simulink model "test"  (R2015b)
settings: Solver=VariableStepAuto  StartTime=0.0  StopTime=10.0  RelTol=1e-3
undefined symbols (not defined in the file or in its folder): etaCmax, etaCmin, m_dot_cCorr, PiC, PiC_at_etaCmax, Q11, Q12, Q22, WcCorr_at_etaCmax
settings Model: Creator=nicgr354  LastModifiedBy=nicgr354

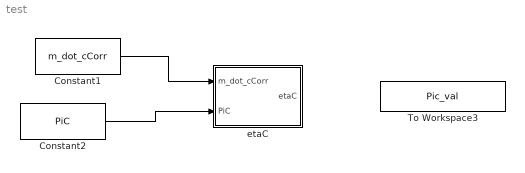
== system test ==
  Constant1 : Constant  Value=m_dot_cCorr
  Constant2 : Constant  Value=PiC
  To Workspace3 : ToWorkspace  VariableName=Pic_val  SampleTime=-1
  etaC : Subsystem
  wires:
  Constant2/1 -> etaC/2(PiC)
  Constant1/1 -> etaC/1(m_dot_cCorr)

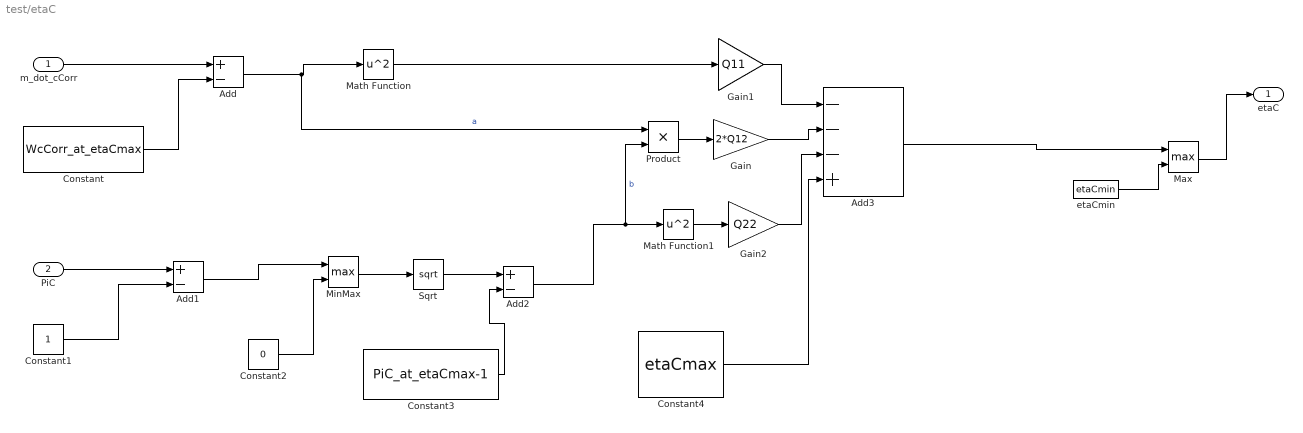
== system test/etaC ==
  m_dot_cCorr : Inport
  PiC : Inport  Port=2
  Add : Sum  Inputs=+-
  Add1 : Sum  Inputs=+-
  Add2 : Sum  Inputs=+-
  Add3 : Sum  Inputs=---+
  Constant : Constant  Value=WcCorr_at_etaCmax
  Constant1 : Constant
  Constant2 : Constant  Value=0
  Constant3 : Constant  Value=PiC_at_etaCmax-1
  Constant4 : Constant  Value=etaCmax
  Gain : Gain  Gain=2*Q12
  Gain1 : Gain  Gain=Q11
  Gain2 : Gain  Gain=Q22
  Math Function : Math  Operator=square  SaturateOnIntegerOverflow=on
  Math Function1 : Math  Operator=square  SaturateOnIntegerOverflow=on
  Max : MinMax  Function=max  Inputs=2
  MinMax : MinMax  Function=max  Inputs=2
  Product : Product
  Sqrt : Sqrt  SaturateOnIntegerOverflow=on
  etaCmin : Constant  Value=etaCmin
  etaC : Outport
  wires:
  PiC/1 -> Add1/1
  m_dot_cCorr/1 -> Add/1
  Max/1 -> etaC/1
  etaCmin/1 -> Max/2
  Add3/1 -> Max/1
  Constant/1 -> Add/2
  Add/1 -> Product/1, Math Function/1  "a"
  Constant1/1 -> Add1/2
  Constant2/1 -> MinMax/2
  Add1/1 -> MinMax/1
  MinMax/1 -> Sqrt/1
  Sqrt/1 -> Add2/1
  Constant3/1 -> Add2/2
  Math Function/1 -> Gain1/1
  Gain1/1 -> Add3/1
  Gain/1 -> Add3/2
  Gain2/1 -> Add3/3
  Add2/1 -> Product/2, Math Function1/1  "b"
  Math Function1/1 -> Gain2/1
  Product/1 -> Gain/1
  Constant4/1 -> Add3/4
